simulink model "part2"  (R2025a)
settings: Solver=ode45  StartTime=0.0  StopTime=25  FixedStep=1  RelTol=1e-3
values from neighbouring files (symbols this model uses):
  A = cases(c).A    [run_S1.m]    (also in run_S12_part2.m = A_list(Ai); assignin('base','A',A))
  amp = cases(c).amp    [run_S1.m]    (also in run_S12_part2.m = 1)
  b1 = 1    [run_S12_part2.m]
  b2 = 1    [run_S12_part2.m]
  freq = cases(c).freq    [run_S1.m]    (also in run_S12_part2.m = 5)
  J1 = 100    [run_S12_part2.m]
  J2 = 1    [run_S12_part2.m]
  k = k_list(kk); assignin('base','k',k)    [run_S12_part2.m]
  theta01 = 0    [run_S12_part2.m]
  theta02 = 0    [run_S12_part2.m]
  useStep = cases(c).useStep    [run_S1.m]    (also in run_S12_part2.m = 1)
  w01 = 0    [run_S12_part2.m]
  w02 = 0    [run_S12_part2.m]
settings Model: Creator=RAJOS  LastModifiedBy=RAJOS

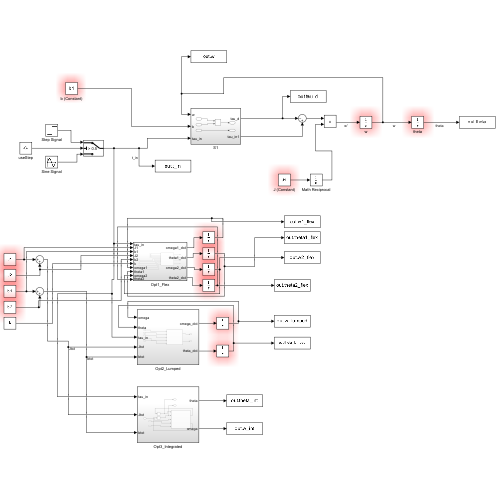
[thumbnail: Simulink's stored preview of the top-level diagram]
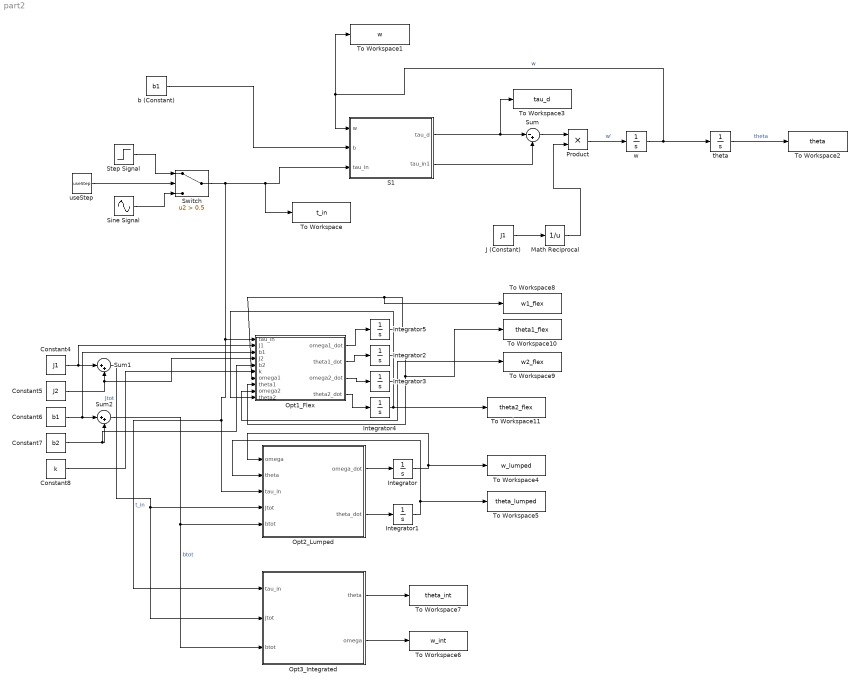
== system part2 ==
  Constant4 : Constant  Value=J1
  Constant5 : Constant  Value=J2
  Constant6 : Constant  Value=b1
  Constant7 : Constant  Value=b2
  Constant8 : Constant  Value=k
  Integrator : Integrator  InitialCondition=w01
  Integrator1 : Integrator  InitialCondition=theta01
  Integrator2 : Integrator  InitialCondition=theta01
  Integrator3 : Integrator  InitialCondition=w02
  Integrator4 : Integrator  InitialCondition=theta02
  Integrator5 : Integrator  InitialCondition=w01
  J (Constant) : Constant  Value=J1
  Math Reciprocal : Math  Operator=reciprocal  SignedPower=on
  Opt1_Flex : Subsystem
  Opt2_Lumped : Subsystem
  Opt3_Integrated : Subsystem
  Product : Product
  S1 : Subsystem
  Sine Signal : Sin  Amplitude=amp  Frequency=freq  SampleTime=0
  Step Signal : Step  Time=0  After=A  SampleTime=0
  Sum : Sum  Inputs=|-+
  Sum1 : Sum  Inputs=|++
  Sum2 : Sum  Inputs=|++
  Switch : Switch  Criteria=u2 > Threshold  Threshold=0.5  SaturateOnIntegerOverflow=off  InputSameDT=off
  To Workspace : ToWorkspace  VariableName=t_in  SampleTime=-1
  To Workspace1 : ToWorkspace  VariableName=w  SampleTime=-1
  To Workspace10 : ToWorkspace  VariableName=theta1_flex  SampleTime=-1
  To Workspace11 : ToWorkspace  VariableName=theta2_flex  SampleTime=-1
  To Workspace2 : ToWorkspace  VariableName=theta  SampleTime=-1
  To Workspace3 : ToWorkspace  VariableName=tau_d  SampleTime=-1
  To Workspace4 : ToWorkspace  VariableName=w_lumped  SampleTime=-1
  To Workspace5 : ToWorkspace  VariableName=theta_lumped  SampleTime=-1
  To Workspace6 : ToWorkspace  VariableName=w_int  SampleTime=-1
  To Workspace7 : ToWorkspace  VariableName=theta_int  SaveFormat=Timeseries  SampleTime=-1
  To Workspace8 : ToWorkspace  VariableName=w1_flex  SampleTime=-1
  To Workspace9 : ToWorkspace  VariableName=w2_flex  SampleTime=-1
  b (Constant) : Constant  Value=b1
  theta : Integrator  InitialCondition=theta01
  useStep : Constant  Value=useStep
  w : Integrator  InitialCondition=w01
  wires:
  Step Signal/1 -> Switch/1
  J (Constant)/1 -> Math Reciprocal/1
  S1/1(tau_d) -> To Workspace3/1, Sum/1
  S1/2(tau_in1) -> Sum/2
  Math Reciprocal/1 -> Product/2
  theta/1 -> To Workspace2/1  "theta"
  Sum/1 -> Product/1
  Sine Signal/1 -> Switch/3
  useStep/1 -> Switch/2
  Product/1 -> w/1  "w'"
  b (Constant)/1 -> S1/2(b)
  Switch/1 -> To Workspace/1, S1/3(tau_in), Opt3_Integrated/1(tau_in), Opt2_Lumped/3(tau_in), Opt1_Flex/1(tau_in)  "t_in"
  w/1 -> To Workspace1/1, S1/1(w), theta/1  "w"
  Opt2_Lumped/1(omega_dot) -> Integrator/1
  Integrator/1 -> Opt2_Lumped/1(omega), To Workspace4/1
  Opt2_Lumped/2(theta_dot) -> Integrator1/1
  Integrator1/1 -> Opt2_Lumped/2(theta), To Workspace5/1
  Sum1/1 -> Opt3_Integrated/2(Jtot), Opt2_Lumped/4(Jtot)  "Jtot"
  Sum2/1 -> Opt3_Integrated/3(btot), Opt2_Lumped/5(btot)  "btot"
  Constant6/1 -> Opt1_Flex/3(b1), Sum2/1
  Constant4/1 -> Opt1_Flex/2(J1), Sum1/1
  Constant5/1 -> Opt1_Flex/4(J2), Sum1/2
  Constant7/1 -> Opt1_Flex/5(b2), Sum2/2
  Constant8/1 -> Opt1_Flex/6(k)
  Opt1_Flex/1(omega1_dot) -> Integrator5/1
  Opt1_Flex/2(theta1_dot) -> Integrator2/1
  Opt1_Flex/3(omega2_dot) -> Integrator3/1
  Opt1_Flex/4(theta2_dot) -> Integrator4/1
  Integrator5/1 -> To Workspace8/1, Opt1_Flex/7(omega1)
  Integrator2/1 -> To Workspace10/1, Opt1_Flex/8(theta1)
  Integrator3/1 -> Opt1_Flex/9(omega2), To Workspace9/1
  Integrator4/1 -> Opt1_Flex/10(theta2), To Workspace11/1
  Opt3_Integrated/1(theta) -> To Workspace7/1
  Opt3_Integrated/2(omega) -> To Workspace6/1

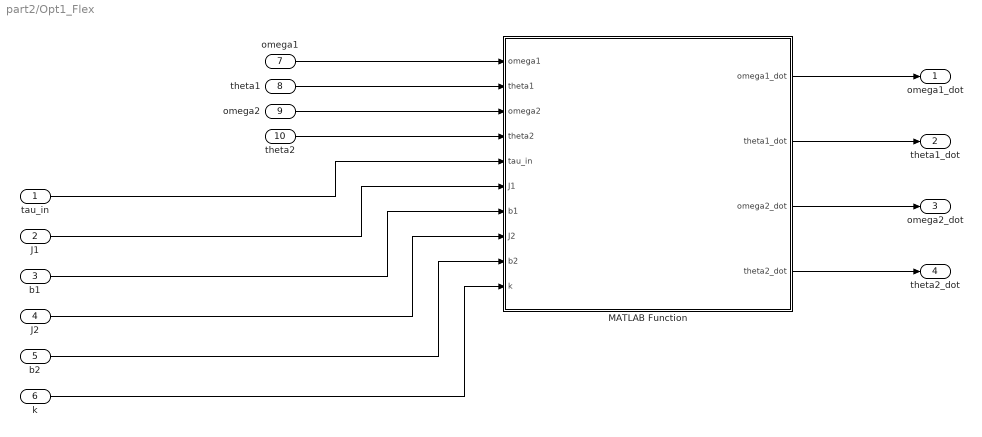
== system part2/Opt1_Flex ==
  tau_in : Inport
  J1 : Inport  Port=2
  b1 : Inport  Port=3
  J2 : Inport  Port=4
  b2 : Inport  Port=5
  k : Inport  Port=6
  omega1 : Inport  Port=7
  theta1 : Inport  Port=8
  omega2 : Inport  Port=9
  theta2 : Inport  Port=10
  MATLAB Function : MATLAB Function  TreatAsAtomicUnit=on
  omega1_dot : Outport
  theta1_dot : Outport  Port=2
  omega2_dot : Outport  Port=3
  theta2_dot : Outport  Port=4
  wires:
  tau_in/1 -> MATLAB Function/5(tau_in)
  J1/1 -> MATLAB Function/6(J1)
  b1/1 -> MATLAB Function/7(b1)
  J2/1 -> MATLAB Function/8(J2)
  b2/1 -> MATLAB Function/9(b2)
  k/1 -> MATLAB Function/10(k)
  omega1/1 -> MATLAB Function/1(omega1)
  theta1/1 -> MATLAB Function/2(theta1)
  omega2/1 -> MATLAB Function/3(omega2)
  theta2/1 -> MATLAB Function/4(theta2)
  MATLAB Function/1(omega1_dot) -> omega1_dot/1
  MATLAB Function/2(theta1_dot) -> theta1_dot/1
  MATLAB Function/3(omega2_dot) -> omega2_dot/1
  MATLAB Function/4(theta2_dot) -> theta2_dot/1

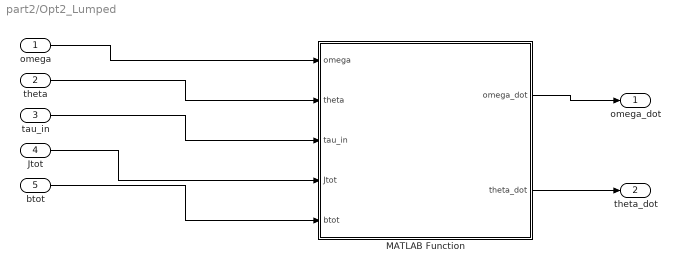
== system part2/Opt2_Lumped ==
  omega : Inport
  theta : Inport  Port=2
  tau_in : Inport  Port=3
  Jtot : Inport  Port=4
  btot : Inport  Port=5
  MATLAB Function : MATLAB Function  TreatAsAtomicUnit=on
  omega_dot : Outport
  theta_dot : Outport  Port=2
  wires:
  omega/1 -> MATLAB Function/1(omega)
  theta/1 -> MATLAB Function/2(theta)
  tau_in/1 -> MATLAB Function/3(tau_in)
  Jtot/1 -> MATLAB Function/4(Jtot)
  btot/1 -> MATLAB Function/5(btot)
  MATLAB Function/1(omega_dot) -> omega_dot/1
  MATLAB Function/2(theta_dot) -> theta_dot/1

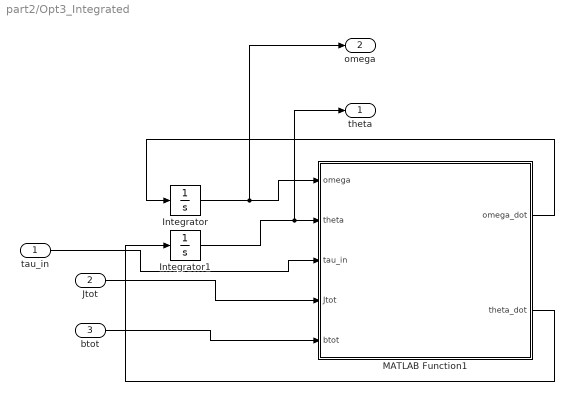
== system part2/Opt3_Integrated ==
  tau_in : Inport
  Jtot : Inport  Port=2
  btot : Inport  Port=3
  Integrator : Integrator  InitialCondition=w01
  Integrator1 : Integrator  InitialCondition=theta01
  MATLAB Function1 : MATLAB Function  TreatAsAtomicUnit=on
  theta : Outport
  omega : Outport  Port=2
  wires:
  Integrator/1 -> omega/1, MATLAB Function1/1(omega)
  Integrator1/1 -> theta/1, MATLAB Function1/2(theta)
  Jtot/1 -> MATLAB Function1/4(Jtot)
  btot/1 -> MATLAB Function1/5(btot)
  tau_in/1 -> MATLAB Function1/3(tau_in)
  MATLAB Function1/1(omega_dot) -> Integrator/1
  MATLAB Function1/2(theta_dot) -> Integrator1/1

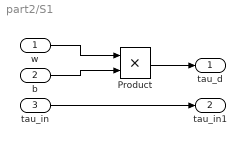
== system part2/S1 ==
  w : Inport
  b : Inport  Port=2
  tau_in : Inport  Port=3
  Product : Product
  tau_d : Outport
  tau_in1 : Outport  Port=2
  wires:
  w/1 -> Product/1
  b/1 -> Product/2
  Product/1 -> tau_d/1
  tau_in/1 -> tau_in1/1

== matlab function part2/Opt2_Lumped/MATLAB Function ==
  data: omega input; omega_dot output; theta input; tau_in input; Jtot input; btot input; theta_dot output
function [omega_dot, theta_dot] = f_S12_combined(omega, theta, tau_in, Jtot, btot)

% Lumped dynamics: Jtot*omega_dot + btot*omega = tau_in
omega_dot = (tau_in - btot*omega)/Jtot;
theta_dot = omega;
end

== matlab function part2/Opt1_Flex/MATLAB Function ==
  data: omega1 input; omega1_dot output; theta1 input; omega2 input; theta2 input; tau_in input; J1 input; b1 input; J2 input; b2 input; k input; theta1_dot output; omega2_dot output; theta2_dot output
function [omega1_dot, theta1_dot, omega2_dot, theta2_dot] = f_S12_flex(omega1, theta1, omega2, theta2, tau_in, J1, b1, J2, b2, k)
% Two inertias with shaft stiffness k
tau_k      = k * (theta1 - theta2);
omega1_dot = (tau_in - b1*omega1 - tau_k) / J1;
theta1_dot = omega1;
omega2_dot = (tau_k - b2*omega2) / J2;
theta2_dot = omega2;
end

== matlab function part2/Opt3_Integrated/MATLAB Function1 ==
  data: omega input; omega_dot output; theta input; tau_in input; Jtot input; btot input; theta_dot output
function [omega_dot, theta_dot] = f_S12_combined(omega, theta, tau_in, Jtot, btot)

% Lumped dynamics: Jtot*omega_dot + btot*omega = tau_in
omega_dot = (tau_in - btot*omega)/Jtot;
theta_dot = omega;
end
